simulink model "RefModel_AeroDyn_Sim"  (R2020b)
settings: Solver=ode1  StartTime=tspan(1)  StopTime=inf  FixedStep=1/sensorFs.imuUpdateFs  RelTol=1e-3  EnableMultiTasking=on
undefined symbols (not defined in the file or in its folder): ACTUATOR_SET, Earth, ENVIRONMENT_SET, F, Light, MIL, sensorFs, SIM_SENSOR_SET, UAVPARAM_SET, WGS84
libraries: simulink x10, aerolibactuator x9, aerolibnav x6, sharedutil x5, shared6dofsys x3, aerolibwind2 x2, aerolibasang x2, aerolibatmos2 x1, aerolibconvert2 x1, aerolibgravity2 x1, aerolibtransform2 x1
(part 2 of 3)

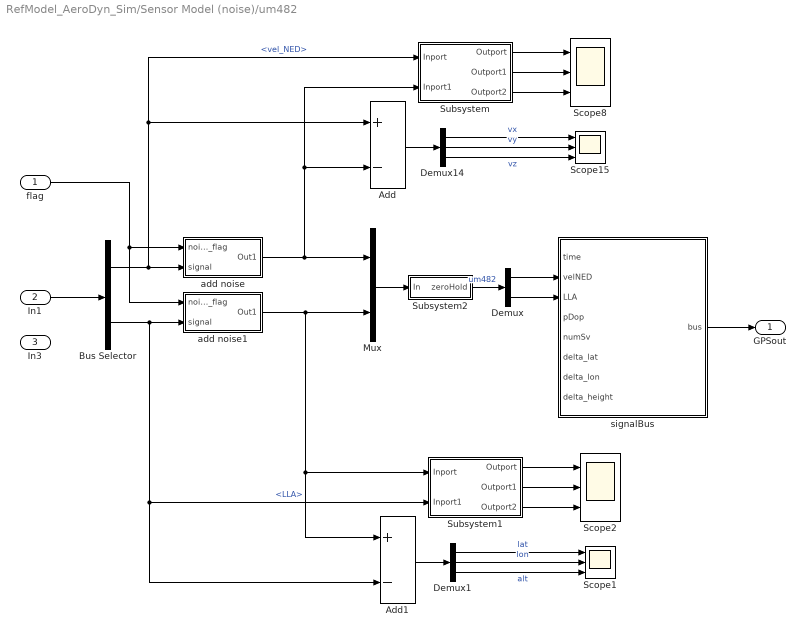
== system RefModel_AeroDyn_Sim/Sensor Model (noise)/um482 ==
  flag : Inport
  In1 : Inport  Port=2
  In3 : Inport  Port=3
  Add : Sum  Inputs=+-
  Add1 : Sum  Inputs=+-
  Bus Selector : BusSelector  OutputSignals=vel_NED,LLA
  Demux : Demux  Outputs=2
  Demux1 : Demux  Outputs=3
  Demux14 : Demux  Outputs=3
  Mux : Mux  Inputs=2
  Scope{1..2,8,15} (4 alike) : Scope  NumInputPorts=3
  Subsystem : Subsystem
  Subsystem1 : Subsystem
  Subsystem2 : Subsystem  mask{sample_freq=sensorFs.gpsUpdateFs}
      mask prompts: sample_freq "采样频率(Hz)"
  add noise : Subsystem
  add noise1 : Subsystem
  signalBus : Subsystem
  GPSout : Outport
  wires:
  In1/1 -> Bus Selector/1
  Bus Selector/2 -> Add1/2, Subsystem1/2(Inport1), add noise1/2(signal)  "<LLA>"
  Bus Selector/1 -> Subsystem/1(Inport), Add/1, add noise/2(signal)  "<vel_NED>"
  add noise/1(Out1) -> Mux/1, Subsystem/2(Inport1), Add/2
  Subsystem/2(Outport1) -> Scope8/2
  Demux14/1 -> Scope15/1  "vx"
  Subsystem/1(Outport) -> Scope8/1
  Subsystem/3(Outport2) -> Scope8/3
  Demux14/2 -> Scope15/2  "vy"
  Add/1 -> Demux14/1
  Demux14/3 -> Scope15/3  "vz"
  Demux1/3 -> Scope1/3  "alt"
  Add1/1 -> Demux1/1
  Demux1/2 -> Scope1/2  "lon"
  Subsystem1/3(Outport2) -> Scope2/3
  Subsystem1/1(Outport) -> Scope2/1
  Demux1/1 -> Scope1/1  "lat"
  Subsystem1/2(Outport1) -> Scope2/2
  add noise1/1(Out1) -> Mux/2, Add1/1, Subsystem1/1(Inport)
  Mux/1 -> Subsystem2/1(In)
  Subsystem2/1(zeroHold) -> Demux/1  "um482"
  Demux/1 -> signalBus/2(velNED)
  Demux/2 -> signalBus/3(LLA)
  signalBus/1(bus) -> GPSout/1
  flag/1 -> add noise1/1(noise_flag), add noise/1(noise_flag)

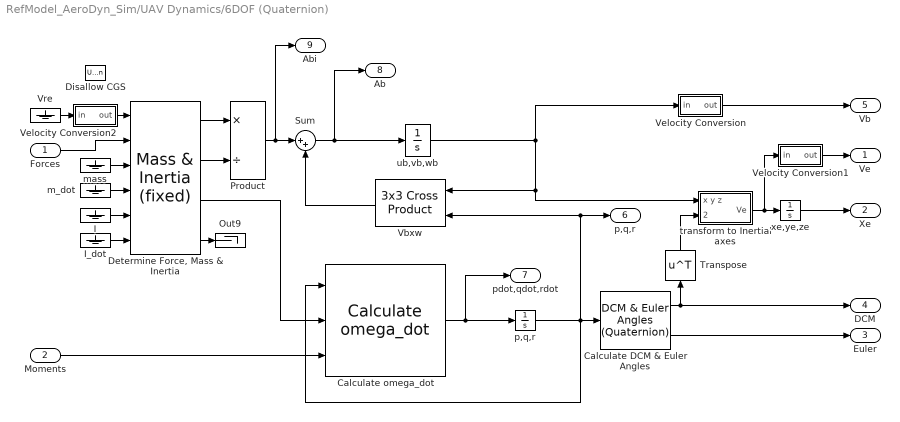
== system RefModel_AeroDyn_Sim/UAV Dynamics/6DOF (Quaternion) ==
  Forces : Inport  Unit=N  PortDimensions=3
  Moments : Inport  Port=2  Unit=N*m  PortDimensions=3
  Calculate DCM & Euler Angles : shared6dofsys/DCM & Euler Angles (Quaternion)  aMode=aMode
      settings: SourceProductBaseCode=AE,PW,MT,UV,VE,VP
  Calculate omega_dot : shared6dofsys/Calculate omega_dot  aMode=aMode
      settings: SourceProductBaseCode=AE,PW,MT,UV,VE,VP
  "Determine Force, Mass & Inertia" : shared6dofsys/Mass & Inertia (fixed)  aMode=aMode
      settings: SourceProductBaseCode=AE,PW,MT,UV,VE,VP
  Disallow CGS : UnitConfiguration  UnitSystemsStr=English,SI,SI (extended)  AllowAllUnitSystems=off
  I : Ground
  I_dot : Ground
  Out9 : Terminator
  Product : Product  Inputs=*/  SaturateOnIntegerOverflow=on  OutDataTypeStr=Inherit: Same as first input
  Sum : Sum  Inputs=|++  SaturateOnIntegerOverflow=on
  Transpose : Math  Operator=transpose  SignedPower=on  SaturateOnIntegerOverflow=on
  Vbxw : sharedutil/3x3 Cross Product  aMode=aMode
      settings: SourceProductBaseCode=AE,PW,MT,UV,VE,VP
  Velocity Conversion : Subsystem
  Velocity Conversion1 : Subsystem
  Velocity Conversion2 : Subsystem
  Vre : Ground
  m_dot : Ground
  mass : Ground
  "p,q,r " : Integrator  InitialCondition=pm_0  ContinuousStateAttributes=pm_statename
  "transform to Inertial axes " : Subsystem  mask(Vector Transformation){}
      mask Display: disp('L_EB')
  ub,vb,wb : Integrator  InitialCondition=Vm_0  ContinuousStateAttributes=Vm_statename
  xe,ye,ze : Integrator  InitialCondition=xme_0  ContinuousStateAttributes=xme_statename
  Ve : Outport  Unit=m/s  VectorParamsAs1DForOutWhenUnconnected=off
  Xe : Outport  Port=2  Unit=m  VectorParamsAs1DForOutWhenUnconnected=off
  Euler : Outport  Port=3  Unit=rad  VectorParamsAs1DForOutWhenUnconnected=off
  DCM : Outport  Port=4  Unit=1  VectorParamsAs1DForOutWhenUnconnected=off
  Vb : Outport  Port=5  Unit=m/s  VectorParamsAs1DForOutWhenUnconnected=off
  p,q,r : Outport  Port=6  Unit=rad/s  VectorParamsAs1DForOutWhenUnconnected=off
  pdot,qdot,rdot : Outport  Port=7  Unit=rad/s^2  VectorParamsAs1DForOutWhenUnconnected=off
  Ab : Outport  Port=8  Unit=m/s^2  VectorParamsAs1DForOutWhenUnconnected=off
  Abi : Outport  Port=9  Unit=m/s^2
  wires:
  Velocity Conversion1/1(out) -> Ve/1
  Sum/1 -> Ab/1, ub,vb,wb/1
  ub,vb,wb/1 -> "transform to Inertial axes "/1(x y z), Vbxw/1, Velocity Conversion/1(in)
  Velocity Conversion/1(out) -> Vb/1
  Velocity Conversion2/1(out) -> "Determine Force, Mass & Inertia"/1
  Vre/1 -> Velocity Conversion2/1(in)
  "Determine Force, Mass & Inertia"/1 -> Product/1
  I_dot/1 -> "Determine Force, Mass & Inertia"/6
  I/1 -> "Determine Force, Mass & Inertia"/5
  Calculate omega_dot/1 -> "p,q,r "/1, pdot,qdot,rdot/1
  "Determine Force, Mass & Inertia"/4 -> Out9/1
  m_dot/1 -> "Determine Force, Mass & Inertia"/4
  "Determine Force, Mass & Inertia"/2 -> Product/2
  mass/1 -> "Determine Force, Mass & Inertia"/3
  Transpose/1 -> "transform to Inertial axes "/2(transform coefficients)
  Calculate DCM & Euler Angles/1 -> Transpose/1, DCM/1
  Product/1 -> Sum/1, Abi/1
  Forces/1 -> "Determine Force, Mass & Inertia"/2
  Moments/1 -> Calculate omega_dot/3
  "p,q,r "/1 -> Calculate omega_dot/1, Calculate DCM & Euler Angles/1, p,q,r/1, Vbxw/2
  "transform to Inertial axes "/1(Ve) -> xe,ye,ze/1, Velocity Conversion1/1(in)
  xe,ye,ze/1 -> Xe/1
  Vbxw/1 -> Sum/2
  Calculate DCM & Euler Angles/2 -> Euler/1
  "Determine Force, Mass & Inertia"/3 -> Calculate omega_dot/2

== system RefModel_AeroDyn_Sim/UAV Dynamics/UAVPARAM ==
  Constant : Constant  Value=UAVPARAM_SET.pressureCenter
  Constant1 : Constant  Value=UAVPARAM_SET.gravityCenter
  Constant2 : Constant  Value=UAVPARAM_SET.S
  Constant3 : Constant  Value=UAVPARAM_SET.meanAerodynamicChord
  Constant4 : Constant  Value=UAVPARAM_SET.wingspan
  Constant5 : Constant  Value=UAVPARAM_SET.mass
  Constant6 : Constant  Value=UAVPARAM_SET.inertia
  pressureCenter : Outport
  gravityCenter : Outport  Port=2
  S : Outport  Port=3
  meanAerodynamicChord : Outport  Port=4
  wingspan : Outport  Port=5
  mass : Outport  Port=6
  inertia : Outport  Port=7
  wires:
  Constant1/1 -> gravityCenter/1  "gravityCenter"
  Constant/1 -> pressureCenter/1  "pressureCenter"
  Constant2/1 -> S/1  "S"
  Constant3/1 -> meanAerodynamicChord/1  "meanAerodynamicChord"
  Constant4/1 -> wingspan/1  "wingspan"
  Constant5/1 -> mass/1  "wingspan"
  Constant6/1 -> inertia/1  "wingspan"

== system RefModel_AeroDyn_Sim/UAV Dynamics/Wind Angle ==
  Vb : Inport  PortDimensions=3
  Vw_body : Inport  Port=2
  rho : Inport  Port=3
  Add : Sum  Inputs=+-
  Dynamic Pressure : aerolibasang/Dynamic Pressure
  "Incidence, Sideslip, & Airspeed" : aerolibasang/Incidence, Sideslip, & Airspeed
  alpha : Outport  VectorParamsAs1DForOutWhenUnconnected=off
  beta : Outport  Port=2  VectorParamsAs1DForOutWhenUnconnected=off
  airspeed : Outport  Port=3  VectorParamsAs1DForOutWhenUnconnected=off
  qbar : Outport  Port=4  VectorParamsAs1DForOutWhenUnconnected=off
  groundSpeed : Outport  Port=5  VectorParamsAs1DForOutWhenUnconnected=off
  wires:
  "Incidence, Sideslip, & Airspeed"/1 -> alpha/1  "alpha"
  "Incidence, Sideslip, & Airspeed"/2 -> beta/1  "beta"
  "Incidence, Sideslip, & Airspeed"/3 -> airspeed/1  "airpseed"
  Vb/1 -> groundSpeed/1, Add/1
  Vw_body/1 -> Add/2
  Add/1 -> Dynamic Pressure/1, "Incidence, Sideslip, & Airspeed"/1
  Dynamic Pressure/1 -> qbar/1  "q"
  rho/1 -> Dynamic Pressure/2

== system RefModel_AeroDyn_Sim/UAV Dynamics/calMagnetic ==
  LLA : Inport
  DCMbe : Inport  Port=2
  Constant : Constant  Value=UAVPARAM_SET.mag_NED
  Demux2 : Demux  Outputs=3
  Display{,1..3} (4 alike) : Display
  Divide2 : Product  Inputs=**  Multiplication=Matrix(*)
  International Geomagnetic Reference Field 12 : aerolibgravity2/International Geomagnetic Reference Field 12  units=Metric (MKS)  time_in=off  month=January  day=1  year=2020  action=None  sv_out=on
      settings: SourceProductBaseCode=AE
  Manual Switch : ManualSwitch  CurrentSetting=0
  Rate Transition : RateTransition  OutPortSampleTime=2
  Rate Transition1 : RateTransition
  Rate Transition2 : RateTransition
  Rate Transition3 : RateTransition
  Reshape : Reshape
  nT to Gs : Gain  Gain=1/1e5
  magBody : Outport  Unit=G
  magNED : Outport  Port=2  Unit=G
  magDec : Outport  Port=3
  wires:
  International Geomagnetic Reference Field 12/1 -> Rate Transition1/1
  DCMbe/1 -> Divide2/1
  Divide2/1 -> Display1/1, Reshape/1
  LLA/1 -> Rate Transition/1
  Reshape/1 -> magBody/1
  Rate Transition/1 -> Demux2/1
  Rate Transition1/1 -> Display2/1, nT to Gs/1
  Manual Switch/1 -> Rate Transition3/1, Divide2/2
  Demux2/3 -> International Geomagnetic Reference Field 12/1
  Demux2/1 -> International Geomagnetic Reference Field 12/2
  Demux2/2 -> International Geomagnetic Reference Field 12/3
  Constant/1 -> Display3/1, Manual Switch/1
  nT to Gs/1 -> Display/1, Manual Switch/2
  International Geomagnetic Reference Field 12/3 -> Rate Transition2/1
  Rate Transition2/1 -> magDec/1
  Rate Transition3/1 -> magNED/1

== system RefModel_AeroDyn_Sim/UAV Dynamics/calSpecificForce ==
  Ftotal : Inport
  DCMbe : Inport  Port=2
  gravity : Inport  Port=3
  Add6 : Sum  Inputs=+-
  Display : Display
  Divide1 : Product  Inputs=**  Multiplication=Matrix(*)
  SFbody : Outport
  wires:
  DCMbe/1 -> Divide1/1
  Divide1/1 -> Display/1, Add6/2
  Add6/1 -> SFbody/1
  Ftotal/1 -> Add6/1
  gravity/1 -> Divide1/2

== system RefModel_AeroDyn_Sim/UAV Dynamics/flat2lla ==
  posNED : Inport
  Constant9 : Constant  Value=UAVPARAM_SET.refloc(3)
  Display10 : Display
  Display9 : Display
  Flat Earth to LLA : aerolibtransform2/Flat Earth to LLA  units=Metric (MKS)  ptype=Earth (WGS84)  F=1/298.257223563  R=6378137  LL0=UAVPARAM_SET.refloc(1:2)  psi=0
  Mux5 : Mux  Inputs=2
  LLA : Outport
  wires:
  Flat Earth to LLA/2 -> Mux5/2, Display10/1
  Constant9/1 -> Flat Earth to LLA/2
  posNED/1 -> Flat Earth to LLA/1
  Flat Earth to LLA/1 -> Mux5/1, Display9/1
  Mux5/1 -> LLA/1

== system RefModel_AeroDyn_Sim/Environment Model/Wind Model/Subsystem ==
  In1 : Inport
  Demux : Demux  Outputs=3
  Mux : Mux  Inputs=3
  Transfer Fcn1 : TransferFcn  Denominator=[0.05 1]
  Transfer Fcn2 : TransferFcn  Denominator=[0.05 1]
  Transfer Fcn3 : TransferFcn  Denominator=[0.05 1]
  Out1 : Outport
  wires:
  Demux/1 -> Transfer Fcn1/1
  Transfer Fcn1/1 -> Mux/1
  Mux/1 -> Out1/1
  Transfer Fcn2/1 -> Mux/2
  In1/1 -> Demux/1
  Demux/2 -> Transfer Fcn2/1
  Transfer Fcn3/1 -> Mux/3
  Demux/3 -> Transfer Fcn3/1

== system RefModel_AeroDyn_Sim/Environment Model/Wind Model/Subsystem1 ==
  In1 : Inport
  Demux : Demux  Outputs=3
  Mux : Mux  Inputs=3
  Transfer Fcn1 : TransferFcn  Denominator=[0.05 1]
  Transfer Fcn2 : TransferFcn  Denominator=[0.05 1]
  Transfer Fcn3 : TransferFcn  Denominator=[0.05 1]
  Out1 : Outport
  wires:
  Demux/3 -> Transfer Fcn3/1
  Transfer Fcn3/1 -> Mux/3
  Demux/2 -> Transfer Fcn2/1
  In1/1 -> Demux/1
  Transfer Fcn2/1 -> Mux/2
  Mux/1 -> Out1/1
  Transfer Fcn1/1 -> Mux/1
  Demux/1 -> Transfer Fcn1/1

== system RefModel_AeroDyn_Sim/Force and Moment/Aero Surface/Get Forces and Moments ==
  q : Inport
  S : Inport  Port=2
  meanAerodynamicChord : Inport  Port=3
  wingspan : Inport  Port=4
  AeroCoeffs : Inport  Port=5
  Bus Selector : BusSelector  OutputSignals=signal2.CD,signal1.CY,signal2.CL
  Bus Selector3 : BusSelector  OutputSignals=signal1.Cl,signal1.Cn
  Bus Selector4 : BusSelector  OutputSignals=signal2.Cm
  Fx_a(Drag) : Product  Inputs=**  SaturateOnIntegerOverflow=on  OutDataTypeStr=Inherit: Same as first input
  Fy_a(Side) : Product  SaturateOnIntegerOverflow=on  OutDataTypeStr=Inherit: Same as first input
  Fz_a(Lift) : Product  SaturateOnIntegerOverflow=on  OutDataTypeStr=Inherit: Same as first input
  Mux : Mux  Inputs=3
  Mux1 : Mux  Inputs=3
  Mx_a : Product  Inputs=3  SaturateOnIntegerOverflow=on  OutDataTypeStr=Inherit: Same as first input
  My_a : Product  Inputs=3  SaturateOnIntegerOverflow=on  OutDataTypeStr=Inherit: Same as first input
  Mz_a : Product  Inputs=3  SaturateOnIntegerOverflow=on  OutDataTypeStr=Inherit: Same as first input
  Product1 : Product  SaturateOnIntegerOverflow=on  OutDataTypeStr=Inherit: Same as first input
  F_aero : Outport  VectorParamsAs1DForOutWhenUnconnected=off
  M_aero : Outport  Port=2  VectorParamsAs1DForOutWhenUnconnected=off
  wires:
  Mx_a/1 -> Mux1/1  "Mx_a"
  Bus Selector/2 -> Fy_a(Side)/1  "<CY>"
  Bus Selector4/1 -> My_a/1  "<Cm>"
  Fx_a(Drag)/1 -> Mux/1  "Fx_a"
  Bus Selector/1 -> Fx_a(Drag)/1  "<CD>"
  AeroCoeffs/1 -> Bus Selector/1, Bus Selector4/1, Bus Selector3/1
  My_a/1 -> Mux1/2  "My_a"
  Fz_a(Lift)/1 -> Mux/3  "Fz_a"
  Mz_a/1 -> Mux1/3  "Mz_a"
  meanAerodynamicChord/1 -> My_a/3
  wingspan/1 -> Mx_a/3, Mz_a/3
  Fy_a(Side)/1 -> Mux/2  "Fy_a"
  Bus Selector3/2 -> Mz_a/1  "<Cn>"
  Bus Selector/3 -> Fz_a(Lift)/1  "<CL>"
  Product1/1 -> Fx_a(Drag)/2, Fy_a(Side)/2, Fz_a(Lift)/2, Mx_a/2, My_a/2, Mz_a/2  "qS"
  Bus Selector3/1 -> Mx_a/1  "<Cl>"
  q/1 -> Product1/1
  S/1 -> Product1/2
  Mux/1 -> F_aero/1
  Mux1/1 -> M_aero/1

== system RefModel_AeroDyn_Sim/Force and Moment/Aero Surface/Lateral Channel ==
  beta : Inport
  alpha : Inport  Port=2
  airspeed : Inport  Port=3
  aileronLeft : Inport  Port=4
  aileronRight : Inport  Port=5
  rudder : Inport  Port=6
  p,q,r : Inport  Port=7
  wingspan : Inport  Port=8
  Add : Sum
  Bus Creator : BusCreator  Inputs=3
  CY : Subsystem
  Cl : Subsystem
  Cn : Subsystem
  Gain : Gain  Gain=1/2
  Lateral : Outport  VectorParamsAs1DForOutWhenUnconnected=off
  wires:
  Cl/1(Cl) -> Bus Creator/2  "Cl"
  p,q,r/1 -> Cn/4(p,q,r), Cl/4(p,q,r)
  airspeed/1 -> Cn/5(Airspeed), CY/3(airspeed), Cl/5(Airspeed)
  rudder/1 -> CY/2(rudder), Cl/3(rudder), Cn/3(rudder)
  Add/1 -> Gain/1
  beta/1 -> Cn/1(beta), Cl/1(beta), CY/1(beta)
  Cn/1(Cn) -> Bus Creator/3  "Cn"
  CY/1(CY) -> Bus Creator/1  "CY"
  Bus Creator/1 -> Lateral/1
  aileronLeft/1 -> Add/1
  aileronRight/1 -> Add/2
  Gain/1 -> Cn/2(aileron), Cl/2(aileron)
  wingspan/1 -> Cn/6(wingspan), Cl/6(wingspan)

== system RefModel_AeroDyn_Sim/Force and Moment/Aero Surface/Longitudinal Channel ==
  beta : Inport
  alpha : Inport  Port=2
  airpseed : Inport  Port=3
  elevator : Inport  Port=4
  p,q,r : Inport  Port=5
  meanAerodynamicChord : Inport  Port=6
  Bus Creator : BusCreator  Inputs=3
  CD : Subsystem
  CL : Subsystem
  Cm : Subsystem
  Longitudinal : Outport  VectorParamsAs1DForOutWhenUnconnected=off
  wires:
  airpseed/1 -> Cm/4(airspeed), CL/3(airspeed), CD/2(airspeed)
  p,q,r/1 -> Cm/3(p,q,r)
  Bus Creator/1 -> Longitudinal/1
  Cm/1(Cm) -> Bus Creator/3  "Cm"
  elevator/1 -> Cm/2(De), CL/2(elevator)
  CL/1(CL) -> Bus Creator/2  "CL"
  CD/1(CD) -> Bus Creator/1  "CD"
  alpha/1 -> CD/1(alpha), Cm/1(alpha), CL/1(alpha)

== system RefModel_AeroDyn_Sim/Force and Moment/Rotor Force/Left Back ==
  tiltRotor : Inport
  tiltGear : Inport  Port=2
  3x3 Cross Product : sharedutil/3x3 Cross Product  aMode=aMode
      settings: SourceProductBaseCode=AE,PW,MT,UV,VE,VP
  Add : Sum  Inputs=+-
  Add1 : Sum
  Add2 : Sum
  Constant : Constant  Value=ACTUATOR_SET.tiltGearLeft.installPosition
  Constant1 : Constant  Value=ACTUATOR_SET.tiltGearLeft.sideAngle
  Constant2 : Constant  Value=UAVPARAM_SET.gravityCenter
  Constant3 : Constant  Value=ACTUATOR_SET.tiltGearLeft.longitudeAngle
  Constant4 : Constant  Value=[1;0;0]
  Display{,1..3} (4 alike) : Display
  Divide : Product  Inputs=**
  Gain : Gain  Gain=-1
  MATLAB Function : MATLAB Function  TreatAsAtomicUnit=on
  Rotor 2814 : Subsystem
  Fb : Outport
  Mb : Outport  Port=2
  wires:
  Rotor 2814/1(pull) -> Divide/2
  Divide/1 -> Display1/1, Fb/1, 3x3 Cross Product/2
  Constant2/1 -> Add/2
  Add/1 -> Display2/1, 3x3 Cross Product/1
  Constant/1 -> Add/1
  Constant4/1 -> MATLAB Function/3(vec0)
  Constant1/1 -> MATLAB Function/1(sideAngle)
  MATLAB Function/1(forceBody) -> Display3/1, Divide/1
  Add1/1 -> MATLAB Function/2(lonAngle)
  Constant3/1 -> Add1/2
  tiltGear/1 -> Gain/1
  tiltRotor/1 -> Rotor 2814/1(pwm)
  3x3 Cross Product/1 -> Add2/1
  Add2/1 -> Display/1, Mb/1
  Rotor 2814/2(torque) -> Add2/2
  Gain/1 -> Add1/1

== system RefModel_AeroDyn_Sim/Force and Moment/Rotor Force/Left Forward ==
  In1 : Inport
  3x3 Cross Product : sharedutil/3x3 Cross Product  aMode=aMode
      settings: SourceProductBaseCode=AE,PW,MT,UV,VE,VP
  Add : Sum  Inputs=+-
  Add1 : Sum
  Constant : Constant  Value=ACTUATOR_SET.verticalRotorLeft.sideAngle
  Constant1 : Constant  Value=ACTUATOR_SET.verticalRotorLeft.installPosition
  Constant2 : Constant  Value=UAVPARAM_SET.gravityCenter
  Constant3 : Constant  Value=ACTUATOR_SET.verticalRotorLeft.longitudeAngle
  Constant4 : Constant  Value=[1;0;0]
  Display{,1..4} (5 alike) : Display
  Divide : Product  Inputs=**
  MATLAB Function : MATLAB Function  TreatAsAtomicUnit=on
  Rotor 5208 : Subsystem
  Fb : Outport
  Mb : Outport  Port=2
  wires:
  Rotor 5208/1(pull) -> Divide/2
  Divide/1 -> 3x3 Cross Product/2, Display2/1, Fb/1
  Constant1/1 -> Add/1
  Add/1 -> Display3/1, 3x3 Cross Product/1
  Constant2/1 -> Add/2
  MATLAB Function/1(forceBody) -> Divide/1, Display/1
  Constant/1 -> MATLAB Function/1(sideAngle)
  Constant3/1 -> MATLAB Function/2(lonAngle)
  Constant4/1 -> MATLAB Function/3(vec0)
  In1/1 -> Rotor 5208/1(pwm)
  Rotor 5208/2(torque) -> Display4/1, Add1/2
  3x3 Cross Product/1 -> Add1/1
  Add1/1 -> Display1/1, Mb/1

== system RefModel_AeroDyn_Sim/Force and Moment/Rotor Force/Right Back ==
  tiltRotor : Inport
  tiltGear : Inport  Port=2
  3x3 Cross Product : sharedutil/3x3 Cross Product  aMode=aMode
      settings: SourceProductBaseCode=AE,PW,MT,UV,VE,VP
  Add : Sum  Inputs=+-
  Add1 : Sum
  Add2 : Sum
  Constant : Constant  Value=ACTUATOR_SET.tiltGearRight.installPosition
  Constant1 : Constant  Value=ACTUATOR_SET.tiltGearRight.sideAngle
  Constant2 : Constant  Value=UAVPARAM_SET.gravityCenter
  Constant3 : Constant  Value=ACTUATOR_SET.tiltGearRight.longitudeAngle
  Constant4 : Constant  Value=[1;0;0]
  Display{,1..3} (4 alike) : Display
  Divide : Product  Inputs=**
  Gain : Gain  Gain=-1
  MATLAB Function : MATLAB Function  TreatAsAtomicUnit=on
  Rotor 2814 : Subsystem
  Fb : Outport
  Mb : Outport  Port=2
  wires:
  Constant3/1 -> Add1/2
  Add1/1 -> MATLAB Function/2(lonAngle)
  MATLAB Function/1(forceBody) -> Divide/1, Display3/1
  Constant1/1 -> MATLAB Function/1(sideAngle)
  Constant4/1 -> MATLAB Function/3(vec0)
  Constant/1 -> Add/1
  Add/1 -> 3x3 Cross Product/1, Display2/1
  Constant2/1 -> Add/2
  Divide/1 -> 3x3 Cross Product/2, Fb/1, Display1/1
  Rotor 2814/1(pull) -> Divide/2
  tiltGear/1 -> Gain/1
  tiltRotor/1 -> Rotor 2814/1(pwm)
  3x3 Cross Product/1 -> Add2/1
  Add2/1 -> Display/1, Mb/1
  Rotor 2814/2(torque) -> Add2/2
  Gain/1 -> Add1/1

== system RefModel_AeroDyn_Sim/Force and Moment/Rotor Force/Right Forward ==
  In1 : Inport
  3x3 Cross Product : sharedutil/3x3 Cross Product  aMode=aMode
      settings: SourceProductBaseCode=AE,PW,MT,UV,VE,VP
  Add : Sum  Inputs=+-
  Add1 : Sum
  Constant : Constant  Value=ACTUATOR_SET.verticalRotorRight.sideAngle
  Constant1 : Constant  Value=ACTUATOR_SET.verticalRotorRight.installPosition
  Constant2 : Constant  Value=UAVPARAM_SET.gravityCenter
  Constant3 : Constant  Value=ACTUATOR_SET.verticalRotorRight.longitudeAngle
  Constant4 : Constant  Value=[1;0;0]
  Display{,1..4} (5 alike) : Display
  Divide : Product  Inputs=**
  MATLAB Function : MATLAB Function  TreatAsAtomicUnit=on
  Rotor 5208 : Subsystem
  Fb : Outport
  Mb : Outport  Port=2
  wires:
  Constant2/1 -> Add/2
  Add/1 -> Display3/1, 3x3 Cross Product/1
  Constant1/1 -> Add/1
  Divide/1 -> Display2/1, Fb/1, 3x3 Cross Product/2
  MATLAB Function/1(forceBody) -> Display/1, Divide/1
  Rotor 5208/1(pull) -> Divide/2
  Constant3/1 -> MATLAB Function/2(lonAngle)
  Constant4/1 -> MATLAB Function/3(vec0)
  Constant/1 -> MATLAB Function/1(sideAngle)
  In1/1 -> Rotor 5208/1(pwm)
  3x3 Cross Product/1 -> Add1/1
  Rotor 5208/2(torque) -> Display4/1, Add1/2
  Add1/1 -> Display1/1, Mb/1

== system RefModel_AeroDyn_Sim/Sensor Model (noise)/Airspeed1/Subsystem ==
  Inport : Inport
  Inport1 : Inport  Port=2
  Mux : Mux  Inputs=2
  Outport : Outport
  wires:
  Inport1/1 -> Mux/2
  Inport/1 -> Mux/1
  Mux/1 -> Outport/1

== system RefModel_AeroDyn_Sim/Sensor Model (noise)/Airspeed1/Subsystem3 ==
  In : Inport
  Compare To Zero : simulink/Logic and Bit Operations/Compare To Zero  relop===  OutDataTypeStr=boolean
  Constant : Constant  Value=1/sample_freq
  Digital Clock : DigitalClock  SampleTime=1/sensorFs.imuUpdateFs
  Math Function : Math  Operator=rem  SaturateOnIntegerOverflow=on
  Scope1 : Scope
  Subsystem : Subsystem
  zeroHold : Outport
  wires:
  Digital Clock/1 -> Math Function/1
  Constant/1 -> Math Function/2
  Math Function/1 -> Compare To Zero/1
  Compare To Zero/1 -> Scope1/1, Subsystem/Enable
  Subsystem/1(Out1) -> zeroHold/1
  In/1 -> Subsystem/1(In1)

== system RefModel_AeroDyn_Sim/Sensor Model (noise)/Airspeed1/add noise1 ==
  noise_flag : Inport
  signal : Inport  Port=2
  Add : Sum
  Add1 : Sum
  Divide : Product  Inputs=**
  Divide1 : Product  Inputs=**
  Random Number : RandomNumber  Seed=22
  bias : Constant  Value=0
  bias1 : Constant  Value=SIM_SENSOR_SET.Airspeed.std_speed
  Out1 : Outport
  wires:
  Random Number/1 -> Divide/1
  Divide/1 -> Add/2
  bias/1 -> Add/1
  bias1/1 -> Divide/2
  signal/1 -> Add1/2
  noise_flag/1 -> Divide1/1
  Divide1/1 -> Add1/1
  Add/1 -> Divide1/2
  Add1/1 -> Out1/1

== system RefModel_AeroDyn_Sim/Sensor Model (noise)/Airspeed1/signalBus ==
  time : Inport
  airspeed : Inport  Port=2
  Data Type Conversion1 : DataTypeConversion
  Data Type Conversion3 : DataTypeConversion
  Out Bus Element : Outport  PortName=airspeed1  Element=time
  Out Bus Element1 : Outport  PortName=airspeed1  Element=airspeed
  wires:
  time/1 -> Data Type Conversion3/1
  airspeed/1 -> Data Type Conversion1/1
  Data Type Conversion3/1 -> Out Bus Element/1
  Data Type Conversion1/1 -> Out Bus Element1/1

== system RefModel_AeroDyn_Sim/Sensor Model (noise)/Baro1/Subsystem ==
  Inport : Inport
  Inport1 : Inport  Port=2
  Mux : Mux  Inputs=2
  Outport : Outport
  wires:
  Mux/1 -> Outport/1
  Inport/1 -> Mux/1
  Inport1/1 -> Mux/2

== system RefModel_AeroDyn_Sim/Sensor Model (noise)/Baro1/Subsystem3 ==
  In : Inport
  Compare To Zero : simulink/Logic and Bit Operations/Compare To Zero  relop===  OutDataTypeStr=boolean
  Constant : Constant  Value=1/sample_freq
  Digital Clock : DigitalClock  SampleTime=1/sensorFs.imuUpdateFs
  Math Function : Math  Operator=rem  SaturateOnIntegerOverflow=on
  Scope1 : Scope
  Subsystem : Subsystem
  zeroHold : Outport
  wires:
  In/1 -> Subsystem/1(In1)
  Subsystem/1(Out1) -> zeroHold/1
  Compare To Zero/1 -> Subsystem/Enable, Scope1/1
  Math Function/1 -> Compare To Zero/1
  Constant/1 -> Math Function/2
  Digital Clock/1 -> Math Function/1

== system RefModel_AeroDyn_Sim/Sensor Model (noise)/Baro1/add noise ==
  noise_flag : Inport
  signal : Inport  Port=2
  Add : Sum
  Add1 : Sum
  Divide : Product  Inputs=**
  Divide1 : Product  Inputs=**
  Random Number : RandomNumber  Seed=21
  bias : Constant  Value=0
  bias1 : Constant  Value=SIM_SENSOR_SET.Baro1.std_alt
  Out1 : Outport
  wires:
  Random Number/1 -> Divide/1
  bias1/1 -> Divide/2
  signal/1 -> Add1/2
  noise_flag/1 -> Divide1/1
  Divide1/1 -> Add1/1
  Add/1 -> Divide1/2
  Divide/1 -> Add/2
  bias/1 -> Add/1
  Add1/1 -> Out1/1

== system RefModel_AeroDyn_Sim/Sensor Model (noise)/Baro1/signalBus ==
  time : Inport
  alt_baro : Inport  Port=2
  Data Type Conversion1 : DataTypeConversion
  Data Type Conversion7 : DataTypeConversion
  Out Bus Element : Outport  PortName=baro1  Element=time
  Out Bus Element1 : Outport  PortName=baro1  Element=alt_baro
  wires:
  alt_baro/1 -> Data Type Conversion7/1
  time/1 -> Data Type Conversion1/1
  Data Type Conversion7/1 -> Out Bus Element1/1
  Data Type Conversion1/1 -> Out Bus Element/1

== system RefModel_AeroDyn_Sim/Sensor Model (noise)/IMU1/Frame Transfer ==
  In1 : Inport
  Constant : Constant  Value=SIM_SENSOR_SET.IMU1.Racc_fromBodyFrameToSensorFrame
  Divide : Product  Inputs=**  Multiplication=Matrix(*)
  Out1 : Outport
  wires:
  Divide/1 -> Out1/1
  In1/1 -> Divide/2
  Constant/1 -> Divide/1

== system RefModel_AeroDyn_Sim/Sensor Model (noise)/IMU1/Frame Transfer1 ==
  In1 : Inport
  Constant : Constant  Value=SIM_SENSOR_SET.IMU1.Racc_fromBodyFrameToSensorFrame
  Divide : Product  Inputs=**  Multiplication=Matrix(*)
  Out1 : Outport
  wires:
  Constant/1 -> Divide/1
  In1/1 -> Divide/2
  Divide/1 -> Out1/1

== system RefModel_AeroDyn_Sim/Sensor Model (noise)/IMU1/Subsystem ==
  Inport : Inport
  Inport1 : Inport  Port=2
  Demux7 : Demux  Outputs=3
  Demux8 : Demux  Outputs=3
  Mux : Mux  Inputs=2
  Mux1 : Mux  Inputs=2
  Mux2 : Mux  Inputs=2
  Outport : Outport
  Outport1 : Outport  Port=2
  Outport2 : Outport  Port=3
  wires:
  Demux7/1 -> Mux/1  "yaw [deg]"
  Demux8/1 -> Mux/2  "yaw [deg]"
  Inport/1 -> Demux7/1
  Mux/1 -> Outport/1
  Demux8/3 -> Mux2/2  "roll [deg]"
  Demux7/2 -> Mux1/1
  Inport1/1 -> Demux8/1
  Mux2/1 -> Outport2/1
  Mux1/1 -> Outport1/1
  Demux8/2 -> Mux1/2  "pitch [deg]"
  Demux7/3 -> Mux2/1  "roll [deg]"

== system RefModel_AeroDyn_Sim/Sensor Model (noise)/IMU1/Subsystem1 ==
  Inport : Inport
  Inport1 : Inport  Port=2
  Demux7 : Demux  Outputs=3
  Demux8 : Demux  Outputs=3
  Mux : Mux  Inputs=2
  Mux1 : Mux  Inputs=2
  Mux2 : Mux  Inputs=2
  Outport : Outport
  Outport1 : Outport  Port=2
  Outport2 : Outport  Port=3
  wires:
  Demux7/3 -> Mux2/1  "roll [deg]"
  Demux8/2 -> Mux1/2  "pitch [deg]"
  Mux1/1 -> Outport1/1
  Mux2/1 -> Outport2/1
  Inport1/1 -> Demux8/1
  Demux7/2 -> Mux1/1
  Demux8/3 -> Mux2/2  "roll [deg]"
  Mux/1 -> Outport/1
  Inport/1 -> Demux7/1
  Demux8/1 -> Mux/2  "yaw [deg]"
  Demux7/1 -> Mux/1  "yaw [deg]"

== system RefModel_AeroDyn_Sim/Sensor Model (noise)/IMU1/Subsystem2 ==
  In : Inport
  Compare To Zero : simulink/Logic and Bit Operations/Compare To Zero  relop===  OutDataTypeStr=boolean
  Constant : Constant  Value=1/sample_freq
  Digital Clock : DigitalClock  SampleTime=1/sensorFs.imuUpdateFs
  Math Function : Math  Operator=rem  SaturateOnIntegerOverflow=on
  Scope1 : Scope
  Subsystem : Subsystem
  zeroHold : Outport
  wires:
  In/1 -> Subsystem/1(In1)
  Subsystem/1(Out1) -> zeroHold/1
  Compare To Zero/1 -> Subsystem/Enable, Scope1/1
  Math Function/1 -> Compare To Zero/1
  Constant/1 -> Math Function/2
  Digital Clock/1 -> Math Function/1

== system RefModel_AeroDyn_Sim/Sensor Model (noise)/IMU1/Subsystem3 ==
  flag : Inport
  <specificForce_Body> : Inport  Port=2
  <w_Body> : Inport  Port=3
  <dw_Body> : Inport  Port=4
  Merge : Merge
  Merge1 : Merge
  NOISE : Subsystem
  NOISE FREE : Subsystem
  Rate Transition : RateTransition  OutPortSampleTime=1/sensorFs.imuUpdateFs
  Switch Case : SwitchCase
  accel : Outport
  Out2 : Outport  Port=2
  wires:
  flag/1 -> Rate Transition/1
  <specificForce_Body>/1 -> NOISE FREE/1(In1), NOISE/1(In1)
  <w_Body>/1 -> NOISE FREE/2(In2), NOISE/2(In2)
  <dw_Body>/1 -> NOISE FREE/3(In3), NOISE/3(In3)
  NOISE/1(accel) -> Merge/1
  NOISE/2(Out2) -> Merge1/1
  Switch Case/1 -> NOISE/Action
  Merge/1 -> accel/1
  NOISE FREE/1(accel) -> Merge/2
  Merge1/1 -> Out2/1
  NOISE FREE/2(Out2) -> Merge1/2
  Rate Transition/1 -> Switch Case/1
  Switch Case/2 -> NOISE FREE/Action

== system RefModel_AeroDyn_Sim/Sensor Model (noise)/IMU1/signalBus ==
  time : Inport
  accel : Inport  Port=2
  gyro : Inport  Port=3
  Data Type Conversion{1..7} (7 alike) : DataTypeConversion
  Demux : Demux  Outputs=3
  Demux1 : Demux  Outputs=3
  Out Bus Element : Outport  PortName=IMU1  Element=time
  Out Bus Element1 : Outport  PortName=IMU1  Element=accel_x
  Out Bus Element2 : Outport  PortName=IMU1  Element=accel_y
  Out Bus Element3 : Outport  PortName=IMU1  Element=accel_z
  Out Bus Element4 : Outport  PortName=IMU1  Element=gyro_x
  Out Bus Element5 : Outport  PortName=IMU1  Element=gyro_y
  Out Bus Element6 : Outport  PortName=IMU1  Element=gyro_z
  wires:
  time/1 -> Data Type Conversion3/1
  Demux/1 -> Data Type Conversion1/1
  Demux/2 -> Data Type Conversion2/1
  Demux/3 -> Data Type Conversion4/1
  Demux1/3 -> Data Type Conversion6/1
  Demux1/2 -> Data Type Conversion5/1
  Demux1/1 -> Data Type Conversion7/1
  accel/1 -> Demux/1
  gyro/1 -> Demux1/1
  Data Type Conversion2/1 -> Out Bus Element2/1
  Data Type Conversion1/1 -> Out Bus Element1/1
  Data Type Conversion3/1 -> Out Bus Element/1
  Data Type Conversion4/1 -> Out Bus Element3/1
  Data Type Conversion5/1 -> Out Bus Element5/1
  Data Type Conversion7/1 -> Out Bus Element4/1
  Data Type Conversion6/1 -> Out Bus Element6/1

== system RefModel_AeroDyn_Sim/Sensor Model (noise)/IMU2/Frame Transfer ==
  In1 : Inport
  Constant : Constant  Value=SIM_SENSOR_SET.IMU2.Racc_fromBodyFrameToSensorFrame
  Divide : Product  Inputs=**  Multiplication=Matrix(*)
  Out1 : Outport
  wires:
  Divide/1 -> Out1/1
  In1/1 -> Divide/2
  Constant/1 -> Divide/1

== system RefModel_AeroDyn_Sim/Sensor Model (noise)/IMU2/Frame Transfer1 ==
  In1 : Inport
  Constant : Constant  Value=SIM_SENSOR_SET.IMU2.Racc_fromBodyFrameToSensorFrame
  Divide : Product  Inputs=**  Multiplication=Matrix(*)
  Out1 : Outport
  wires:
  Constant/1 -> Divide/1
  In1/1 -> Divide/2
  Divide/1 -> Out1/1

== system RefModel_AeroDyn_Sim/Sensor Model (noise)/IMU2/Subsystem ==
  Inport : Inport
  Inport1 : Inport  Port=2
  Demux7 : Demux  Outputs=3
  Demux8 : Demux  Outputs=3
  Mux : Mux  Inputs=2
  Mux1 : Mux  Inputs=2
  Mux2 : Mux  Inputs=2
  Outport : Outport
  Outport1 : Outport  Port=2
  Outport2 : Outport  Port=3
  wires:
  Demux7/1 -> Mux/1  "yaw [deg]"
  Demux8/1 -> Mux/2  "yaw [deg]"
  Inport/1 -> Demux7/1
  Mux/1 -> Outport/1
  Demux8/3 -> Mux2/2  "roll [deg]"
  Demux7/2 -> Mux1/1
  Inport1/1 -> Demux8/1
  Mux2/1 -> Outport2/1
  Mux1/1 -> Outport1/1
  Demux8/2 -> Mux1/2  "pitch [deg]"
  Demux7/3 -> Mux2/1  "roll [deg]"

== system RefModel_AeroDyn_Sim/Sensor Model (noise)/IMU2/Subsystem1 ==
  Inport : Inport
  Inport1 : Inport  Port=2
  Demux7 : Demux  Outputs=3
  Demux8 : Demux  Outputs=3
  Mux : Mux  Inputs=2
  Mux1 : Mux  Inputs=2
  Mux2 : Mux  Inputs=2
  Outport : Outport
  Outport1 : Outport  Port=2
  Outport2 : Outport  Port=3
  wires:
  Demux7/3 -> Mux2/1  "roll [deg]"
  Demux8/2 -> Mux1/2  "pitch [deg]"
  Mux1/1 -> Outport1/1
  Mux2/1 -> Outport2/1
  Inport1/1 -> Demux8/1
  Demux7/2 -> Mux1/1
  Demux8/3 -> Mux2/2  "roll [deg]"
  Mux/1 -> Outport/1
  Inport/1 -> Demux7/1
  Demux8/1 -> Mux/2  "yaw [deg]"
  Demux7/1 -> Mux/1  "yaw [deg]"

== system RefModel_AeroDyn_Sim/Sensor Model (noise)/IMU2/Subsystem2 ==
  In : Inport
  Compare To Zero : simulink/Logic and Bit Operations/Compare To Zero  relop===  OutDataTypeStr=boolean
  Constant : Constant  Value=1/sample_freq
  Digital Clock : DigitalClock  SampleTime=1/sensorFs.imuUpdateFs
  Math Function : Math  Operator=rem  SaturateOnIntegerOverflow=on
  Scope1 : Scope
  Subsystem : Subsystem
  zeroHold : Outport
  wires:
  In/1 -> Subsystem/1(In1)
  Subsystem/1(Out1) -> zeroHold/1
  Compare To Zero/1 -> Subsystem/Enable, Scope1/1
  Math Function/1 -> Compare To Zero/1
  Constant/1 -> Math Function/2
  Digital Clock/1 -> Math Function/1

== system RefModel_AeroDyn_Sim/Sensor Model (noise)/IMU2/Subsystem3 ==
  flag : Inport
  <specificForce_Body> : Inport  Port=2
  <w_Body> : Inport  Port=3
  <dw_Body> : Inport  Port=4
  Merge : Merge
  Merge1 : Merge
  NOISE : Subsystem
  NOISE FREE : Subsystem
  Rate Transition : RateTransition  OutPortSampleTime=1/sensorFs.imuUpdateFs
  Switch Case : SwitchCase
  accel : Outport
  Out2 : Outport  Port=2
  wires:
  flag/1 -> Rate Transition/1
  <specificForce_Body>/1 -> NOISE FREE/1(In1), NOISE/1(In1)
  <w_Body>/1 -> NOISE FREE/2(In2), NOISE/2(In2)
  <dw_Body>/1 -> NOISE FREE/3(In3), NOISE/3(In3)
  NOISE/1(accel) -> Merge/1
  NOISE/2(Out2) -> Merge1/1
  Switch Case/1 -> NOISE/Action
  Merge/1 -> accel/1
  NOISE FREE/1(accel) -> Merge/2
  Merge1/1 -> Out2/1
  NOISE FREE/2(Out2) -> Merge1/2
  Rate Transition/1 -> Switch Case/1
  Switch Case/2 -> NOISE FREE/Action

== system RefModel_AeroDyn_Sim/Sensor Model (noise)/IMU2/signalBus ==
  time : Inport
  accel : Inport  Port=2
  gyro : Inport  Port=3
  Data Type Conversion{1..7} (7 alike) : DataTypeConversion
  Demux : Demux  Outputs=3
  Demux1 : Demux  Outputs=3
  Out Bus Element : Outport  PortName=IMU1  Element=time
  Out Bus Element1 : Outport  PortName=IMU1  Element=accel_x
  Out Bus Element2 : Outport  PortName=IMU1  Element=accel_y
  Out Bus Element3 : Outport  PortName=IMU1  Element=accel_z
  Out Bus Element4 : Outport  PortName=IMU1  Element=gyro_x
  Out Bus Element5 : Outport  PortName=IMU1  Element=gyro_y
  Out Bus Element6 : Outport  PortName=IMU1  Element=gyro_z
  wires:
  time/1 -> Data Type Conversion3/1
  Demux/1 -> Data Type Conversion1/1
  Demux/2 -> Data Type Conversion2/1
  Demux/3 -> Data Type Conversion4/1
  Demux1/3 -> Data Type Conversion6/1
  Demux1/2 -> Data Type Conversion5/1
  Demux1/1 -> Data Type Conversion7/1
  accel/1 -> Demux/1
  gyro/1 -> Demux1/1
  Data Type Conversion2/1 -> Out Bus Element2/1
  Data Type Conversion1/1 -> Out Bus Element1/1
  Data Type Conversion3/1 -> Out Bus Element/1
  Data Type Conversion4/1 -> Out Bus Element3/1
  Data Type Conversion5/1 -> Out Bus Element5/1
  Data Type Conversion7/1 -> Out Bus Element4/1
  Data Type Conversion6/1 -> Out Bus Element6/1

== system RefModel_AeroDyn_Sim/Sensor Model (noise)/IMU3/Frame Transfer ==
  In1 : Inport
  Constant : Constant  Value=SIM_SENSOR_SET.IMU3.Racc_fromBodyFrameToSensorFrame
  Divide : Product  Inputs=**  Multiplication=Matrix(*)
  Out1 : Outport
  wires:
  Divide/1 -> Out1/1
  In1/1 -> Divide/2
  Constant/1 -> Divide/1

== system RefModel_AeroDyn_Sim/Sensor Model (noise)/IMU3/Frame Transfer1 ==
  In1 : Inport
  Constant : Constant  Value=SIM_SENSOR_SET.IMU3.Racc_fromBodyFrameToSensorFrame
  Divide : Product  Inputs=**  Multiplication=Matrix(*)
  Out1 : Outport
  wires:
  Constant/1 -> Divide/1
  In1/1 -> Divide/2
  Divide/1 -> Out1/1

== system RefModel_AeroDyn_Sim/Sensor Model (noise)/IMU3/Subsystem ==
  Inport : Inport
  Inport1 : Inport  Port=2
  Demux7 : Demux  Outputs=3
  Demux8 : Demux  Outputs=3
  Mux : Mux  Inputs=2
  Mux1 : Mux  Inputs=2
  Mux2 : Mux  Inputs=2
  Outport : Outport
  Outport1 : Outport  Port=2
  Outport2 : Outport  Port=3
  wires:
  Demux7/3 -> Mux2/1  "roll [deg]"
  Demux8/2 -> Mux1/2  "pitch [deg]"
  Mux1/1 -> Outport1/1
  Mux2/1 -> Outport2/1
  Inport1/1 -> Demux8/1
  Demux7/2 -> Mux1/1
  Demux8/3 -> Mux2/2  "roll [deg]"
  Mux/1 -> Outport/1
  Inport/1 -> Demux7/1
  Demux8/1 -> Mux/2  "yaw [deg]"
  Demux7/1 -> Mux/1  "yaw [deg]"

== system RefModel_AeroDyn_Sim/Sensor Model (noise)/IMU3/Subsystem1 ==
  Inport : Inport
  Inport1 : Inport  Port=2
  Demux7 : Demux  Outputs=3
  Demux8 : Demux  Outputs=3
  Mux : Mux  Inputs=2
  Mux1 : Mux  Inputs=2
  Mux2 : Mux  Inputs=2
  Outport : Outport
  Outport1 : Outport  Port=2
  Outport2 : Outport  Port=3
  wires:
  Demux7/1 -> Mux/1  "yaw [deg]"
  Demux8/1 -> Mux/2  "yaw [deg]"
  Inport/1 -> Demux7/1
  Mux/1 -> Outport/1
  Demux8/3 -> Mux2/2  "roll [deg]"
  Demux7/2 -> Mux1/1
  Inport1/1 -> Demux8/1
  Mux2/1 -> Outport2/1
  Mux1/1 -> Outport1/1
  Demux8/2 -> Mux1/2  "pitch [deg]"
  Demux7/3 -> Mux2/1  "roll [deg]"

== system RefModel_AeroDyn_Sim/Sensor Model (noise)/IMU3/Subsystem2 ==
  In : Inport
  Compare To Zero : simulink/Logic and Bit Operations/Compare To Zero  relop===  OutDataTypeStr=boolean
  Constant : Constant  Value=1/sample_freq
  Digital Clock : DigitalClock  SampleTime=1/sensorFs.imuUpdateFs
  Math Function : Math  Operator=rem  SaturateOnIntegerOverflow=on
  Scope1 : Scope
  Subsystem : Subsystem
  zeroHold : Outport
  wires:
  In/1 -> Subsystem/1(In1)
  Subsystem/1(Out1) -> zeroHold/1
  Compare To Zero/1 -> Subsystem/Enable, Scope1/1
  Math Function/1 -> Compare To Zero/1
  Constant/1 -> Math Function/2
  Digital Clock/1 -> Math Function/1

== system RefModel_AeroDyn_Sim/Sensor Model (noise)/IMU3/Subsystem3 ==
  flag : Inport
  <specificForce_Body> : Inport  Port=2
  <w_Body> : Inport  Port=3
  <dw_Body> : Inport  Port=4
  Merge : Merge
  Merge1 : Merge
  NOISE : Subsystem
  NOISE FREE : Subsystem
  Rate Transition : RateTransition  OutPortSampleTime=1/sensorFs.imuUpdateFs
  Switch Case : SwitchCase
  accel : Outport
  Out2 : Outport  Port=2
  wires:
  Switch Case/2 -> NOISE FREE/Action
  Rate Transition/1 -> Switch Case/1
  NOISE FREE/2(Out2) -> Merge1/2
  Merge1/1 -> Out2/1
  NOISE FREE/1(accel) -> Merge/2
  Merge/1 -> accel/1
  Switch Case/1 -> NOISE/Action
  NOISE/2(Out2) -> Merge1/1
  NOISE/1(accel) -> Merge/1
  <dw_Body>/1 -> NOISE FREE/3(In3), NOISE/3(In3)
  <w_Body>/1 -> NOISE FREE/2(In2), NOISE/2(In2)
  <specificForce_Body>/1 -> NOISE FREE/1(In1), NOISE/1(In1)
  flag/1 -> Rate Transition/1

== system RefModel_AeroDyn_Sim/Sensor Model (noise)/IMU3/signalBus ==
  time : Inport
  accel : Inport  Port=2
  gyro : Inport  Port=3
  Data Type Conversion{1..7} (7 alike) : DataTypeConversion
  Demux : Demux  Outputs=3
  Demux1 : Demux  Outputs=3
  Out Bus Element : Outport  PortName=IMU1  Element=time
  Out Bus Element1 : Outport  PortName=IMU1  Element=accel_x
  Out Bus Element2 : Outport  PortName=IMU1  Element=accel_y
  Out Bus Element3 : Outport  PortName=IMU1  Element=accel_z
  Out Bus Element4 : Outport  PortName=IMU1  Element=gyro_x
  Out Bus Element5 : Outport  PortName=IMU1  Element=gyro_y
  Out Bus Element6 : Outport  PortName=IMU1  Element=gyro_z
  wires:
  Data Type Conversion6/1 -> Out Bus Element6/1
  Data Type Conversion7/1 -> Out Bus Element4/1
  Data Type Conversion5/1 -> Out Bus Element5/1
  Data Type Conversion4/1 -> Out Bus Element3/1
  Data Type Conversion3/1 -> Out Bus Element/1
  Data Type Conversion1/1 -> Out Bus Element1/1
  Data Type Conversion2/1 -> Out Bus Element2/1
  gyro/1 -> Demux1/1
  accel/1 -> Demux/1
  Demux1/1 -> Data Type Conversion7/1
  Demux1/2 -> Data Type Conversion5/1
  Demux1/3 -> Data Type Conversion6/1
  Demux/3 -> Data Type Conversion4/1
  Demux/2 -> Data Type Conversion2/1
  Demux/1 -> Data Type Conversion1/1
  time/1 -> Data Type Conversion3/1

== system RefModel_AeroDyn_Sim/Sensor Model (noise)/Mag1/BodyFrame to MagFrame ==
  In1 : Inport
  Constant : Constant  Value=SIM_SENSOR_SET.Mag1.R_fromBodyFrameToSensorFrame
  Divide : Product  Inputs=**  Multiplication=Matrix(*)
  Out1 : Outport
  wires:
  In1/1 -> Divide/2
  Constant/1 -> Divide/1
  Divide/1 -> Out1/1

== system RefModel_AeroDyn_Sim/Sensor Model (noise)/Mag1/Subsystem ==
  Inport : Inport
  Inport1 : Inport  Port=2
  Demux7 : Demux  Outputs=3
  Demux8 : Demux  Outputs=3
  Mux : Mux  Inputs=2
  Mux1 : Mux  Inputs=2
  Mux2 : Mux  Inputs=2
  Outport : Outport
  Outport1 : Outport  Port=2
  Outport2 : Outport  Port=3
  wires:
  Demux7/1 -> Mux/1  "yaw [deg]"
  Demux8/1 -> Mux/2  "yaw [deg]"
  Inport/1 -> Demux7/1
  Mux/1 -> Outport/1
  Demux8/3 -> Mux2/2  "roll [deg]"
  Demux7/2 -> Mux1/1
  Inport1/1 -> Demux8/1
  Mux2/1 -> Outport2/1
  Mux1/1 -> Outport1/1
  Demux8/2 -> Mux1/2  "pitch [deg]"
  Demux7/3 -> Mux2/1  "roll [deg]"

== system RefModel_AeroDyn_Sim/Sensor Model (noise)/Mag1/Subsystem9 ==
  In : Inport
  Compare To Zero : simulink/Logic and Bit Operations/Compare To Zero  relop===  OutDataTypeStr=boolean
  Constant : Constant  Value=1/sample_freq
  Digital Clock : DigitalClock  SampleTime=1/sensorFs.imuUpdateFs
  Math Function : Math  Operator=rem  SaturateOnIntegerOverflow=on
  Scope : Scope  NumInputPorts=3
  Scope1 : Scope
  Subsystem : Subsystem
  Zero-Order Hold : ZeroOrderHold
  zeroHold : Outport
  wires:
  Digital Clock/1 -> Math Function/1
  Constant/1 -> Math Function/2
  Math Function/1 -> Compare To Zero/1
  Compare To Zero/1 -> Subsystem/Enable, Scope1/1
  Subsystem/1(Out1) -> Scope/1, zeroHold/1
  In/1 -> Scope/2, Zero-Order Hold/1, Subsystem/1(In1)
  Zero-Order Hold/1 -> Scope/3

== system RefModel_AeroDyn_Sim/Sensor Model (noise)/Mag1/add noise ==
  noise_flag : Inport
  signal : Inport  Port=2
  Add : Sum
  Add1 : Sum
  Divide : Product  Inputs=**
  Divide1 : Product  Inputs=**
  Random Number : RandomNumber  Seed=[12,13,14]
  bias : Constant  Value=SIM_SENSOR_SET.Mag1.mag_bias
  bias1 : Constant  Value=SIM_SENSOR_SET.Mag1.std_mag
  Out1 : Outport
  wires:
  signal/1 -> Add1/2
  Random Number/1 -> Divide/1
  Divide/1 -> Add/2
  bias/1 -> Add/1
  bias1/1 -> Divide/2
  Add1/1 -> Out1/1
  Add/1 -> Divide1/2
  Divide1/1 -> Add1/1
  noise_flag/1 -> Divide1/1

== system RefModel_AeroDyn_Sim/Sensor Model (noise)/Mag1/signalBus ==
  time : Inport
  mag : Inport  Port=2
  Data Type Conversion{,1..3} (4 alike) : DataTypeConversion
  Demux : Demux  Outputs=3
  Out Bus Element : Outport  PortName=mag1  Element=time
  Out Bus Element1 : Outport  PortName=mag1  Element=mag_x
  Out Bus Element2 : Outport  PortName=mag1  Element=mag_y
  Out Bus Element3 : Outport  PortName=mag1  Element=mag_z
  wires:
  Demux/1 -> Data Type Conversion1/1
  time/1 -> Data Type Conversion/1
  Demux/2 -> Data Type Conversion2/1
  Demux/3 -> Data Type Conversion3/1
  mag/1 -> Demux/1
  Data Type Conversion/1 -> Out Bus Element/1
  Data Type Conversion1/1 -> Out Bus Element1/1
  Data Type Conversion2/1 -> Out Bus Element2/1
  Data Type Conversion3/1 -> Out Bus Element3/1

== system RefModel_AeroDyn_Sim/Sensor Model (noise)/Mag2/BodyFrame to MagFrame ==
  In1 : Inport
  Constant : Constant  Value=SIM_SENSOR_SET.Mag1.R_fromBodyFrameToSensorFrame
  Divide : Product  Inputs=**  Multiplication=Matrix(*)
  Out1 : Outport
  wires:
  Divide/1 -> Out1/1
  Constant/1 -> Divide/1
  In1/1 -> Divide/2

== system RefModel_AeroDyn_Sim/Sensor Model (noise)/Mag2/Subsystem ==
  Inport : Inport
  Inport1 : Inport  Port=2
  Demux7 : Demux  Outputs=3
  Demux8 : Demux  Outputs=3
  Mux : Mux  Inputs=2
  Mux1 : Mux  Inputs=2
  Mux2 : Mux  Inputs=2
  Outport : Outport
  Outport1 : Outport  Port=2
  Outport2 : Outport  Port=3
  wires:
  Demux7/3 -> Mux2/1  "roll [deg]"
  Demux8/2 -> Mux1/2  "pitch [deg]"
  Mux1/1 -> Outport1/1
  Mux2/1 -> Outport2/1
  Inport1/1 -> Demux8/1
  Demux7/2 -> Mux1/1
  Demux8/3 -> Mux2/2  "roll [deg]"
  Mux/1 -> Outport/1
  Inport/1 -> Demux7/1
  Demux8/1 -> Mux/2  "yaw [deg]"
  Demux7/1 -> Mux/1  "yaw [deg]"

== system RefModel_AeroDyn_Sim/Sensor Model (noise)/Mag2/Subsystem9 ==
  In : Inport
  Compare To Zero : simulink/Logic and Bit Operations/Compare To Zero  relop===  OutDataTypeStr=boolean
  Constant : Constant  Value=1/sample_freq
  Digital Clock : DigitalClock  SampleTime=1/sensorFs.imuUpdateFs
  Math Function : Math  Operator=rem  SaturateOnIntegerOverflow=on
  Scope : Scope  NumInputPorts=3
  Scope1 : Scope
  Subsystem : Subsystem
  Zero-Order Hold : ZeroOrderHold
  zeroHold : Outport
  wires:
  Zero-Order Hold/1 -> Scope/3
  In/1 -> Subsystem/1(In1), Zero-Order Hold/1, Scope/2
  Subsystem/1(Out1) -> zeroHold/1, Scope/1
  Compare To Zero/1 -> Scope1/1, Subsystem/Enable
  Math Function/1 -> Compare To Zero/1
  Constant/1 -> Math Function/2
  Digital Clock/1 -> Math Function/1

== system RefModel_AeroDyn_Sim/Sensor Model (noise)/Mag2/add noise ==
  noise_flag : Inport
  signal : Inport  Port=2
  Add : Sum
  Add1 : Sum
  Divide : Product  Inputs=**
  Divide1 : Product  Inputs=**
  Random Number : RandomNumber  Seed=[12,13,14]
  bias : Constant  Value=SIM_SENSOR_SET.Mag2.mag_bias
  bias1 : Constant  Value=SIM_SENSOR_SET.Mag2.std_mag
  Out1 : Outport
  wires:
  noise_flag/1 -> Divide1/1
  Divide1/1 -> Add1/1
  Add/1 -> Divide1/2
  Add1/1 -> Out1/1
  bias1/1 -> Divide/2
  bias/1 -> Add/1
  Divide/1 -> Add/2
  Random Number/1 -> Divide/1
  signal/1 -> Add1/2

== system RefModel_AeroDyn_Sim/Sensor Model (noise)/Mag2/signalBus ==
  time : Inport
  mag : Inport  Port=2
  Data Type Conversion{,1..3} (4 alike) : DataTypeConversion
  Demux : Demux  Outputs=3
  Out Bus Element : Outport  PortName=mag1  Element=time
  Out Bus Element1 : Outport  PortName=mag1  Element=mag_x
  Out Bus Element2 : Outport  PortName=mag1  Element=mag_y
  Out Bus Element3 : Outport  PortName=mag1  Element=mag_z
  wires:
  Data Type Conversion3/1 -> Out Bus Element3/1
  Data Type Conversion2/1 -> Out Bus Element2/1
  Data Type Conversion1/1 -> Out Bus Element1/1
  Data Type Conversion/1 -> Out Bus Element/1
  mag/1 -> Demux/1
  Demux/3 -> Data Type Conversion3/1
  Demux/2 -> Data Type Conversion2/1
  time/1 -> Data Type Conversion/1
  Demux/1 -> Data Type Conversion1/1

== system RefModel_AeroDyn_Sim/Sensor Model (noise)/Radar1/Subsystem ==
  Inport : Inport
  Inport1 : Inport  Port=2
  Mux : Mux  Inputs=2
  Outport : Outport
  wires:
  Mux/1 -> Outport/1
  Inport/1 -> Mux/1
  Inport1/1 -> Mux/2

== system RefModel_AeroDyn_Sim/Sensor Model (noise)/Radar1/Subsystem3 ==
  In : Inport
  Compare To Zero : simulink/Logic and Bit Operations/Compare To Zero  relop===  OutDataTypeStr=boolean
  Constant : Constant  Value=1/sample_freq
  Digital Clock : DigitalClock  SampleTime=1/sensorFs.imuUpdateFs
  Math Function : Math  Operator=rem  SaturateOnIntegerOverflow=on
  Scope1 : Scope
  Subsystem : Subsystem
  zeroHold : Outport
  wires:
  In/1 -> Subsystem/1(In1)
  Subsystem/1(Out1) -> zeroHold/1
  Compare To Zero/1 -> Subsystem/Enable, Scope1/1
  Math Function/1 -> Compare To Zero/1
  Constant/1 -> Math Function/2
  Digital Clock/1 -> Math Function/1

== system RefModel_AeroDyn_Sim/Sensor Model (noise)/Radar1/add noise1 ==
  noise_flag : Inport
  signal : Inport  Port=2
  Add : Sum
  Add1 : Sum
  Divide : Product  Inputs=**
  Divide1 : Product  Inputs=**
  Random Number : RandomNumber  Seed=22
  bias : Constant  Value=0
  bias1 : Constant  Value=SIM_SENSOR_SET.Radar1.std_range
  Out1 : Outport
  wires:
  bias1/1 -> Divide/2
  bias/1 -> Add/1
  Divide/1 -> Add/2
  Random Number/1 -> Divide/1
  signal/1 -> Add1/2
  noise_flag/1 -> Divide1/1
  Divide1/1 -> Add1/1
  Add/1 -> Divide1/2
  Add1/1 -> Out1/1

== system RefModel_AeroDyn_Sim/Sensor Model (noise)/Radar1/radar1 ==
  time : Inport
  SNR : Inport  Port=2
  Flag : Inport  Port=3
  Range : Inport  Port=4
  Data Type Conversion{1..4} (4 alike) : DataTypeConversion
  Out Bus Element : Outport  PortName=radar1  Element=time
  Out Bus Element1 : Outport  PortName=radar1  Element=SNR
  Out Bus Element2 : Outport  PortName=radar1  Element=Flag
  Out Bus Element3 : Outport  PortName=radar1  Element=Range
  wires:
  SNR/1 -> Data Type Conversion1/1
  time/1 -> Data Type Conversion3/1
  Flag/1 -> Data Type Conversion2/1
  Range/1 -> Data Type Conversion4/1
  Data Type Conversion3/1 -> Out Bus Element/1
  Data Type Conversion1/1 -> Out Bus Element1/1
  Data Type Conversion2/1 -> Out Bus Element2/1
  Data Type Conversion4/1 -> Out Bus Element3/1

== system RefModel_AeroDyn_Sim/Sensor Model (noise)/Ublox1/Subsystem ==
  Inport : Inport
  Inport1 : Inport  Port=2
  Demux7 : Demux  Outputs=3
  Demux8 : Demux  Outputs=3
  Mux : Mux  Inputs=2
  Mux1 : Mux  Inputs=2
  Mux2 : Mux  Inputs=2
  Outport : Outport
  Outport1 : Outport  Port=2
  Outport2 : Outport  Port=3
  wires:
  Demux7/1 -> Mux/1  "yaw [deg]"
  Demux8/1 -> Mux/2  "yaw [deg]"
  Inport/1 -> Demux7/1
  Mux/1 -> Outport/1
  Demux8/3 -> Mux2/2  "roll [deg]"
  Demux7/2 -> Mux1/1
  Inport1/1 -> Demux8/1
  Mux2/1 -> Outport2/1
  Mux1/1 -> Outport1/1
  Demux8/2 -> Mux1/2  "pitch [deg]"
  Demux7/3 -> Mux2/1  "roll [deg]"

== system RefModel_AeroDyn_Sim/Sensor Model (noise)/Ublox1/Subsystem1 ==
  Inport : Inport
  Inport1 : Inport  Port=2
  Demux7 : Demux  Outputs=3
  Demux8 : Demux  Outputs=3
  Mux : Mux  Inputs=2
  Mux1 : Mux  Inputs=2
  Mux2 : Mux  Inputs=2
  Outport : Outport
  Outport1 : Outport  Port=2
  Outport2 : Outport  Port=3
  wires:
  Demux7/3 -> Mux2/1  "roll [deg]"
  Demux8/2 -> Mux1/2  "pitch [deg]"
  Mux1/1 -> Outport1/1
  Mux2/1 -> Outport2/1
  Inport1/1 -> Demux8/1
  Demux7/2 -> Mux1/1
  Demux8/3 -> Mux2/2  "roll [deg]"
  Mux/1 -> Outport/1
  Inport/1 -> Demux7/1
  Demux8/1 -> Mux/2  "yaw [deg]"
  Demux7/1 -> Mux/1  "yaw [deg]"

== system RefModel_AeroDyn_Sim/Sensor Model (noise)/Ublox1/Subsystem2 ==
  In : Inport
  Compare To Zero : simulink/Logic and Bit Operations/Compare To Zero  relop===  OutDataTypeStr=boolean
  Constant : Constant  Value=1/sample_freq
  Digital Clock : DigitalClock  SampleTime=1/sensorFs.imuUpdateFs
  Math Function : Math  Operator=rem  SaturateOnIntegerOverflow=on
  Scope1 : Scope
  Subsystem : Subsystem
  zeroHold : Outport
  wires:
  Digital Clock/1 -> Math Function/1
  Constant/1 -> Math Function/2
  Math Function/1 -> Compare To Zero/1
  Compare To Zero/1 -> Scope1/1, Subsystem/Enable
  Subsystem/1(Out1) -> zeroHold/1
  In/1 -> Subsystem/1(In1)

== system RefModel_AeroDyn_Sim/Sensor Model (noise)/Ublox1/add noise ==
  noise_flag : Inport
  signal : Inport  Port=2
  Add : Sum
  Add1 : Sum
  Divide : Product  Inputs=**
  Divide1 : Product  Inputs=**
  Random Number : RandomNumber  Seed=[18,19,20]
  bias : Constant  Value=[0,0,0]
  bias1 : Constant  Value=SIM_SENSOR_SET.Ublox1.std_gpsvel
  Out1 : Outport
  wires:
  signal/1 -> Add1/2
  Random Number/1 -> Divide/1
  Divide/1 -> Add/2
  bias/1 -> Add/1
  bias1/1 -> Divide/2
  Add/1 -> Divide1/2
  Divide1/1 -> Add1/1
  noise_flag/1 -> Divide1/1
  Add1/1 -> Out1/1
